simulink model "flightControlSystem"  (R2024b)
settings: Solver=ode3  StartTime=0  StopTime=TFinal  FixedStep=Ts  RelTol=1e-3  EnableMultiTasking=on
undefined symbols (not defined in the file): codertarget, Controller, DiscIntNeverNeededParam, Discrete, Estimator, g, init, Sensors, strel, Time, Ts, var_acc_angle_N, var_bias_gyr_N, var_gyro_p_N, Vehicle
libraries: simulink x40, slpidlib x4, ctrlSharedLib x4, sharedtransform x3, visionmorphops x2, parrotlib x1
(part 3 of 3)

== matlab function flightControlSystem/Control System/Path Planning/MATLAB Function5 ==
  data: prev_deriv_term input; deriv_term output; err_derivative input; change_flag input; prev_counter input; prev_hold_flag input; sample_time input; hold_duration input; deriv_gain input; step_counter output; hold_flag output
function [deriv_term, step_counter, hold_flag] = compute_derivative_term( ...
    prev_deriv_term, err_derivative, change_flag, prev_counter, prev_hold_flag, ...
    sample_time, hold_duration, deriv_gain)
% Computes the derivative component of the path control for the X-axis.
%
% Inputs:
% - prev_deriv_term  : previous derivative term used in planning
% - err_derivative   : current derivative of the error (pixels/frame)
% - change_flag      : indicates a change in the sign/magnitude of error
% - prev_counter     : counter value from previous cycle
% - prev_hold_flag   : hold flag from previous cycle
% - sample_time      : controller sample period
% - hold_duration    : time duration to keep the derivative term active
% - deriv_gain       : multiplier for derivative term
%
% Outputs:
% - deriv_term       : updated derivative contribution
% - step_counter     : updated counter value
% - hold_flag        : double-type flag (1 if derivative term is held)

    % Calculate the number of samples to hold the derivative term
    persistent hold_steps
    if isempty(hold_steps)
        hold_steps = round(hold_duration / sample_time);
    end

    % Default outputs
    hold_flag = 0;  % force as double
    step_counter = 0;
    deriv_term = 0;

    % Start hold if change detected and counter reset
    if change_flag && prev_counter == 0
        hold_flag = 1;
    end

    % If in hold phase (either previously or just triggered now)
    if prev_hold_flag || hold_flag
        if prev_counter >= hold_steps
            % End hold after set time
            step_counter = 0;
            hold_flag = 0;
        else
            % Continue hold and update counter
            step_counter = prev_counter + 1;
            hold_flag = 1;
        end

        % Compute derivative term
        deriv_term = err_derivative * deriv_gain;

        % If derivative goes to zero abruptly, keep previous value
        if deriv_term == 0 && prev_deriv_term ~= 0
            deriv_term = prev_deriv_term;
        end
    end
end

== matlab function flightControlSystem/Control System/Path Planning/MATLAB Function4 ==
  data: err_x input; total_norm_error output; err_y input; end_marker_detected input; prev_norm_error input; current_norm_error output
function [total_norm_error, current_norm_error] = error_function( ...
    err_x, err_y, end_marker_detected, prev_norm_error)
% Calculates the Euclidean error between the drone's center of gravity (CoG)
% and the midpoint of the detected end marker.
%
% Inputs:
% - err_x: displacement along the x-axis from CoG to end marker center.
% - err_y: displacement along the y-axis from CoG to end marker center.
% - end_marker_detected: logical flag, true if end marker is currently found.
% - prev_norm_error: previously stored norm error value.
%
% Outputs:
% - total_norm_error: cumulative norm error, including the previous value.
% - current_norm_error: norm error at the current time step.

% If end marker is present, compute Euclidean distance
if end_marker_detected
    % Compute current norm of error
    current_norm_error = hypot(err_x, err_y);
    
    % Include the previous error value
    total_norm_error = prev_norm_error + current_norm_error;
else
    % Assign a large fixed value when no marker is detected
    large_error_value = 100; % must be greater than MAX_ERROR_LANDING
    current_norm_error = large_error_value;
    total_norm_error = large_error_value;
end

== stateflow chart flightControlSystem/Control System/Path Planning/Chart4 ==
  state LANDING
    entry:
    z_planned=0;
    flag_end_marker_to_controller=1;
  state TRACKING
    entry:
    z_planned=-1.1;
    flag_end_marker_to_controller=0;
  state IDLE
  (default) -> IDLE
  IDLE -> TRACKING : [flag_track==1]
  TRACKING -> LANDING : [flag_end_marker==1&&norm_error<=MAX_ERROR_LANDING]
  data: flag_track input; norm_error input; flag_end_marker_to_controller output; z_planned output; MAX_ERROR_LANDING constant double =5; flag_end_marker input

== matlab function flightControlSystem/Image Processing System/MATLAB Function1 ==
  data: flag_track input; out output
function out = flag_stabilizer(flag_track)
  %#codegen
  persistent count
  if isempty(count)
    count = uint32(0);
  end

  if count < 10
    count = count + 1;
    out = true;            % <— logical-ok
  else
    out = flag_track;      % <— also logical
  end
end

== matlab function flightControlSystem/Image Processing System/Wavepoint Follower ==
  data: binaryFrame input; prevXRef input; prevYRef input; errY output; prevTrackFlag input; rMin input; rMax input; fovRatio input; centerX input; centerY input; errX output; laneAngle output; trackDetected output
function [errY, errX, laneAngle, trackDetected] = ...
    lane_error_estimator(binaryFrame, prevXRef, prevYRef, prevTrackFlag, ...
    rMin, rMax, fovRatio, centerX, centerY)
% This function estimates horizontal (X) and vertical (Y) pixel offsets
% between the drone’s center of gravity (CoG) and a lane point ahead
% using a circular "crown" mask search region.
%
% Inputs:
%   binaryFrame   - binary image (1 = lane pixel, 0 = background)
%   prevXRef      - previous X offset to lane
%   prevYRef      - previous Y offset to lane
%   prevTrackFlag - whether lane was detected in last frame (true/false)
%   rMin, rMax    - inner & outer radius of crown (pixels)
%   fovRatio      - portion of the crown (radians divisor)
%   centerX, centerY - CoG pixel coordinates
%
% Outputs:
%   errY          - pixel offset along Y-axis from CoG to lane point
%   errX          - pixel offset along X-axis from CoG to lane point
%   laneAngle     - estimated lane orientation (radians)
%   trackDetected - true if lane is detected, false otherwise

% --- Persistent storage for pixel stats ---
persistent sumX sumY numPixels
if isempty(sumX), sumX = 0; end
if isempty(sumY), sumY = 0; end
if isempty(numPixels), numPixels = 0; end

% --- Lane heading estimation based on last reference point ---
laneAngle = atan2(-prevXRef, prevYRef);
laneAngle = mod(laneAngle, 2*pi);

% --- Pixel search ---
if prevTrackFlag
    % If lane was previously found, search only in front-facing arc
    for px = (centerX - rMax):(centerX + rMax)
        for py = (centerY - rMax):(centerY + rMax)
            
            radius = sqrt((px - (centerX - 0.5))^2 + (py - (centerY - 0.5))^2);
            if radius >= rMin && radius <= rMax
                
                dx = px - (centerX - 0.5);
                dy = py - (centerY - 0.5);
                pointAngle = mod(atan2(dx, dy), 2*pi);

                upperBound = mod(laneAngle + (pi / fovRatio), 2*pi);
                lowerBound = mod(laneAngle - (pi / fovRatio), 2*pi);

                % Check if pixel lies in FOV arc
                if (upperBound < lowerBound && ...
                    ((pointAngle >= lowerBound && pointAngle <= 2*pi) || ...
                     (pointAngle >= 0 && pointAngle <= upperBound))) || ...
                   (upperBound >= lowerBound && ...
                    (pointAngle >= lowerBound && pointAngle <= upperBound))

                    if binaryFrame(px, py) == 1
                        numPixels = numPixels + 1;
                        sumX = sumX + px;
                        sumY = sumY + py;
                    end
                end
            end
        end
    end
else
    % First-time or lost tracking: search full crown
    for px = (centerX - rMax):(centerX + rMax)
        for py = (centerY - rMax):(centerY + rMax)
            
            radius = sqrt((px - (centerX - 0.5))^2 + (py - (centerY - 0.5))^2);
            if radius >= rMin && radius <= rMax
                if binaryFrame(px, py) == 1
                    numPixels = numPixels + 1;
                    sumX = sumX + px;
                    sumY = sumY + py;
                end
            end
        end
    end
end

% --- Compute reference offsets ---
if numPixels > 0
    refX = -(round(sumX / numPixels) - centerX);
    refY =  (round(sumY / numPixels) - centerY);
else
    refX = NaN;
    refY = NaN;
end

% --- Handle no-lane-detected case ---
if isnan(refX)
    errX = 0;
    xDetected = false;
else
    errX = refX;
    xDetected = true;
end

if isnan(refY)
    errY = 0;
    yDetected = false;
else
    errY = refY;
    yDetected = true;
end

% --- Final track detection flag ---
trackDetected = xDetected || yDetected;

% --- Reset accumulators ---
sumX = 0;
sumY = 0;
numPixels = 0;

end

== matlab function flightControlSystem/Control System/Controller/Position Controller/Position error transformation (Earth to Body frame) ==
  data: yaw input; xy_err_earth input; xy_err_body output
function xy_err_body = fcn(yaw,xy_err_earth)

transformation = [cos(yaw), sin(yaw); -sin(yaw),  cos(yaw)];
xy_err_body = transformation * xy_err_earth;


end

== stateflow chart flightControlSystem/Image Processing System/Chart ==
  state TAKE_OFF
    entry:flag=1;
  state ON_TRACK
    entry:flag=1;
  state OFF_TRACK
    entry:flag=0;
  (default) -> TAKE_OFF
  TAKE_OFF -> ON_TRACK : [flag_track==1]
  ON_TRACK -> OFF_TRACK : [flag_track==0]
  data: flag_track input; flag output

== matlab function flightControlSystem/Image Processing System/MATLAB Function ==
  data: error_x_end_marker output; error_y_end_marker output; flag_end_marker output; binary input; flag input; FRAME_SIZE_WIDTH input; FRAME_SIZE_HEIGHT input; COG_Y input; COG_X input
function [error_x_end_marker, error_y_end_marker, flag_end_marker] = end_marker_detector(binary,flag, ...
    FRAME_SIZE_WIDTH, FRAME_SIZE_HEIGHT, COG_Y, COG_X)
% The MATLAB function computes the errors along the x- and y-axis between
% the drone COG and the middle of the lane. The end marker is detected by 
% using a disk kernel. This function is active only when the drone has 
% arrived at the end of the path.
%
%
% Inputs:
% - binary: binarized frame obtained as the convolution with a disk kernel
% - x_ref_prev: previous value of the tracking point along the x-axis of 
% the track line. It is used as a reference for tracking the path.
% - y_ref_prev: previous value of the tracking point along the y-axis of 
% the track line. It is used as a reference for tracking the path. 
% - flag_track_prev: previous value assumed by the flag variablle, i.e., 
% the previous state of the drone (over the track / not over the track).
%
%
% Outputs:
% - error_y_end_marker: error between the CoG of the drone and a point of the 
% lane in the forward direction along the y-axis. It is expressed in
% pixels.
% - error_x_end_maker: error between the CoG of the drone and a point of the 
% lane in the forward direction along the x-axis. It is expressed in pixels. 
% - flag_end_marker: it is TURE if the Image Processing System detects 
% the end marker.
% - yaw: heading angle of the lane in the image plane.
%
%
%Parameters:
% - COG_X: position of the drone CoG along x-axis of the reference frame.
% - COG_Y: position of the drone CoG along y-axis of the reference frame.
% - FRAME_SIZE_WIDTH: width of the frame.
% - FRAME_SIZE_HEIGHT: height of the frame.

persistent column_accumulator
persistent count_pixel
persistent row_accumulator


if isempty(column_accumulator)
    column_accumulator = 0;
end

if isempty(count_pixel)
    count_pixel = 0;
end

if isempty(row_accumulator)
    row_accumulator = 0;
end

flag_track = flag;


% check if the track is ended
if ~flag_track

    for i=1:FRAME_SIZE_HEIGHT

        for j=1:FRAME_SIZE_WIDTH

            %check all the pixel belonging to the end marker
            if binary(i,j)==1
                count_pixel = count_pixel +1;
                column_accumulator = column_accumulator + j;
                row_accumulator = row_accumulator + i;

            end

        end
    end
    
    if count_pixel ~= 0
        flag_end_marker=1;
        center_x = round(row_accumulator/count_pixel);
        center_y = round(column_accumulator/count_pixel);
    else
        flag_end_marker=0;
        center_x=1;
        center_y=1;
    end

else
    
    center_x = 0;
    center_y = 0;
    flag_end_marker = 0;

end

% Calculate the medium point of the end marker
error_x_end_marker = -(center_x - COG_X);
error_y_end_marker = (center_y - COG_Y);

% reset of the persistent variables
count_pixel = 0;
column_accumulator = 0;
row_accumulator = 0;

output = [error_x_end_marker, error_y_end_marker, flag_end_marker];

end

== matlab function flightControlSystem/Control System/Path Planning/MATLAB Function ==
  data: altitude input; ppReadyFlag output; lowLimit input; highLimit input; waitForHover input
function ppReadyFlag = check_hover_band(altitude, lowLimit, highLimit, waitForHover)
% Determines whether the path planner can be enabled based on altitude range.
%
% Inputs:
%   altitude     - Estimated altitude of the drone (m)
%   lowLimit     - Minimum acceptable hover height (m)
%   highLimit    - Maximum acceptable hover height (m)
%   waitForHover - 0 = require altitude band check, 1 = skip altitude check
%
% Output:
%   ppReadyFlag  - Logical (1/0), true if planner can be activated

    if waitForHover == 0
        % Enable only if altitude lies within the allowed range
        if altitude <= lowLimit && altitude >= highLimit
            ppReadyFlag = 1;
        else
            ppReadyFlag = 0;
        end
    else
        % Skip altitude requirement — always ready
        ppReadyFlag = 1;
    end
end

== matlab function flightControlSystem/Control System/Path Planning/MATLAB Function1 ==
  data: trackX input; trackY input; endX input; endY input; endFlag input; hoverFlag input; errX output; errY output
function [errX, errY] = select_error_source(trackX, trackY, endX, endY, endFlag, hoverFlag)
% Chooses which error signals (tracking or end-marker) should drive
% the drone’s motion, depending on flight status and detections.
%
% Inputs:
%   trackX, trackY - Lane tracking errors (pixels)
%   endX, endY     - End-marker tracking errors (pixels)
%   endFlag        - True if end marker is detected
%   hoverFlag      - True if drone is airborne
%
% Outputs:
%   errX, errY     - Chosen control errors (pixels)

    if hoverFlag
        % If drone is airborne, choose between lane or end marker errors
        if endFlag
            errX = endX;
            errY = endY;
        else
            errX = trackX;
            errY = trackY;
        end
    else
        % If drone is not flying, no error correction needed
        errX = 0;
        errY = 0;
    end
end
